simulink model "sschdlexThreePhaseRectifierExample"  (R2023b)
settings: Solver=FixedStepDiscrete  StartTime=0.0  StopTime=0.025  RelTol=1e-6  AbsTol=1e-6
libraries: fl_lib x19, nesl_utility x11
settings Model: DataTypeOverride=Off  Creator=The MathWorks, Inc.  LastModifiedBy=The MathWorks, Inc.
settings SolverCC: AutoScaleAbsTol=off  AlgebraicLoopSolver=TrustRegion
settings DataIOCC: SaveOutput=off  SignalLogging=off  DSMLogging=off  SaveTime=off  ReturnWorkspaceOutputs=off
settings OptimizationCC: BlockReduction=off  ConditionallyExecuteInputs=off  DefaultParameterBehavior=Inlined
settings DebuggingCC: AlgebraicLoopMsg=error  SingleTaskRateTransMsg=error  UnconnectedInputMsg=warning  UnconnectedOutputMsg=warning  UnconnectedLineMsg=warning  PregeneratedLibrarySubsystemCodeDiagnostic=none  ArithmeticOperatorsInVariantConditions=warning
settings HardwareCC: ProdBitPerPointer=32  ProdBitPerSizeT=32  ProdBitPerPtrDiffT=32  ProdLargestAtomicFloat=None  ProdIntDivRoundTo=Undefined  ProdEndianess=Unspecified  ProdWordSize=32  ProdHWDeviceType=ASIC/FPGA->ASIC/FPGA  TargetBitPerPointer=64  TargetBitPerSizeT=64  TargetBitPerPtrDiffT=64  TargetLongLongMode=on  TargetIntDivRoundTo=Zero  TargetEndianess=LittleEndian  TargetWordSize=64  TargetHWDeviceType=Custom Processor->MATLAB Host Computer  ProdEqTarget=off
settings ModelReferenceCC: EnableRefExpFcnMdlSchedulingChecks=on
settings SFSimCC: SimUseLocalCustomCode=off  CustomCodeUndefinedFunction=UseInterfaceOnly
settings RTWCC: RTWUseLocalCustomCode=off
settings CodeAppCC: StateflowObjectComments=on
settings SimscapeCC: SimscapeNormalizeSystem=off  SimscapeNominalValues="[{\"value\":\"10\",\"unit\":\"V\"},{\"value\":\"1\",\"unit\":\"A\"},{\"value\":\"10\",\"unit\":\"N*m\"},{\"value\":\"10\",\"unit\":\"bar\"},{\"value\":\"100\",\"unit\":\"kJ/kg\"},{\"value\":\"1\",\"unit\":\"kW\"},{\"value\":\"300\",\"unit\":\"K\"},{\"value\":\"100\",\"unit\":\"cm^3/s\"},{\"value\":\"1\",\"unit\":\"kN\"},{\"value\":\"1\",\"unit\":\"g/cm^3\"},{\"value\":\"1\",\"unit\":\"l\"},{\"value\":\"1\",\"unit\":\"cm^2\"},{\"value\":\"60\",\"unit\":\"Hz\"}]"  SimscapeLogType=all  SimscapeLogDataHistory=10000

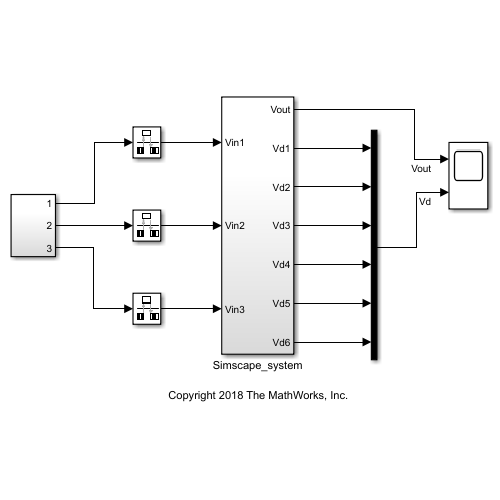
[thumbnail: Simulink's stored preview of the top-level diagram]
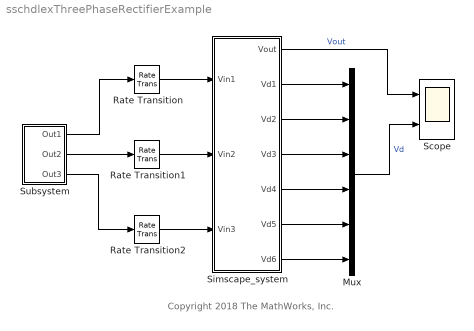
== system sschdlexThreePhaseRectifierExample ==
  note: Copyright 2018 The MathWorks, Inc.
  Mux : Mux  Inputs=6
  Rate Transition : RateTransition
  Rate Transition1 : RateTransition
  Rate Transition2 : RateTransition
  Scope : Scope  NumInputPorts=2
  Simscape_system : Subsystem
  Subsystem : Subsystem
  wires:
  Simscape_system/2(Vd1) -> Mux/1
  Simscape_system/3(Vd2) -> Mux/2
  Simscape_system/4(Vd3) -> Mux/3
  Simscape_system/5(Vd4) -> Mux/4
  Simscape_system/6(Vd5) -> Mux/5
  Simscape_system/7(Vd6) -> Mux/6
  Subsystem/1(Out1) -> Rate Transition/1
  Subsystem/2(Out2) -> Rate Transition1/1
  Subsystem/3(Out3) -> Rate Transition2/1
  Rate Transition/1 -> Simscape_system/1(Vin1)
  Rate Transition1/1 -> Simscape_system/2(Vin2)
  Rate Transition2/1 -> Simscape_system/3(Vin3)
  Simscape_system/1(Vout) -> Scope/1  "Vout"
  Mux/1 -> Scope/2  "Vd"

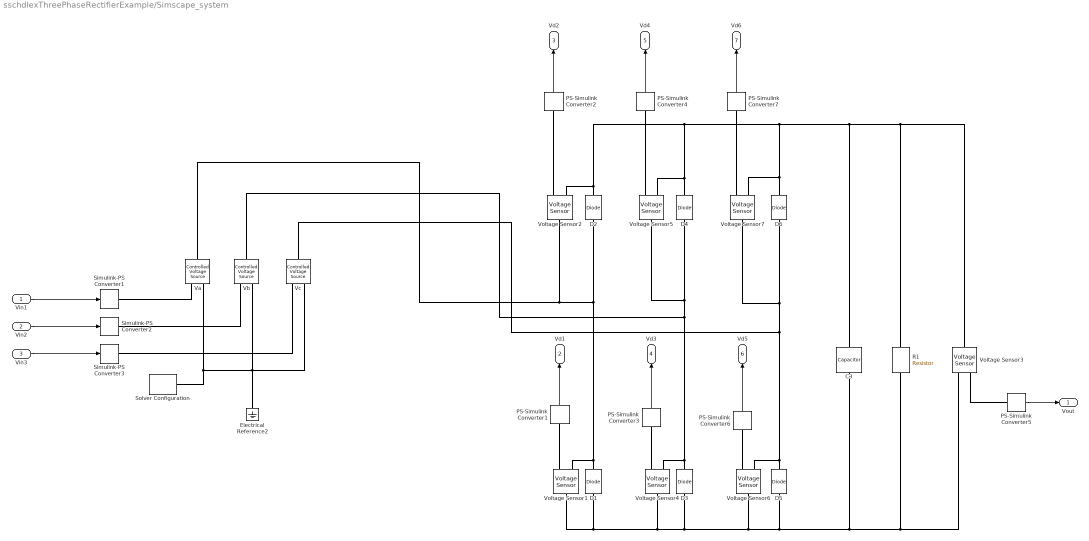
== system sschdlexThreePhaseRectifierExample/Simscape_system ==
  Vin1 : Inport
  Vin2 : Inport  Port=2
  Vin3 : Inport  Port=3
  C3 : fl_lib/Electrical/Electrical Elements/Capacitor  c=10e-3 F  r=1e-6 Ohm  g=0 1/Ohm  i_specify=off  i_priority=None  i=0 A  i_nominal_specify=off  i_nominal_unit=A  i_nominal_value=1  v_specify=off  v_priority=None  v=0 V  v_nominal_specify=off  v_nominal_unit=V  v_nominal_value=1  vc_specify=on  vc_priority=High  vc=150 V  vc_nominal_specify=off  vc_nominal_unit=V  vc_nominal_value=1
  D{1..6} (6 alike) : fl_lib/Electrical/Electrical Elements/Diode  Vf=0.8 V  Ron=0.001 Ohm  Goff=1e-5 1/Ohm  i_specify=off  i_priority=None  i=0 A  i_nominal_specify=off  i_nominal_unit=A  i_nominal_value=1  v_specify=off  v_priority=None  v=0 V  v_nominal_specify=off  v_nominal_unit=V  v_nominal_value=1
  Electrical Reference2 : fl_lib/Electrical/Electrical Elements/Electrical Reference
  PS-Simulink Converter{1..7} (7 alike) : nesl_utility/PS-Simulink Converter  PhysicalDomain=network_engine_domain  SubClassName=ps_output  LeftPortType=input  RightPortType=output  PseudoPeriodic=off  Frequencies=[]  Unit=1  AffineConversion=off
  R1 : fl_lib/Electrical/Electrical Elements/Resistor  R=1 Ohm  i_specify=off  i_priority=None  i=0 A  i_nominal_specify=off  i_nominal_unit=A  i_nominal_value=1  v_specify=off  v_priority=None  v=0 V  v_nominal_specify=off  v_nominal_unit=V  v_nominal_value=1
  Simulink-PS Converter1 : nesl_utility/Simulink-PS Converter  PhysicalDomain=network_engine_domain  SubClassName=ps_input  LeftPortType=input  RightPortType=output  PseudoPeriodic=off  Frequencies=[]  NoiseDistribution=none  NoiseParameters=[]  Unit=1  AffineConversion=off  FilteringAndDerivatives=zero  SimscapeFilterOrder=1  InputFilterTimeConstant=0.001  UdotUserProvided=1
  Simulink-PS Converter2 : nesl_utility/Simulink-PS Converter  PhysicalDomain=network_engine_domain  SubClassName=ps_input  LeftPortType=input  RightPortType=output  PseudoPeriodic=off  Frequencies=[]  NoiseDistribution=none  NoiseParameters=[]  Unit=1  AffineConversion=off  FilteringAndDerivatives=zero  SimscapeFilterOrder=1  InputFilterTimeConstant=0.001  UdotUserProvided=1
  Simulink-PS Converter3 : nesl_utility/Simulink-PS Converter  PhysicalDomain=network_engine_domain  SubClassName=ps_input  LeftPortType=input  RightPortType=output  PseudoPeriodic=off  Frequencies=[]  NoiseDistribution=none  NoiseParameters=[]  Unit=1  AffineConversion=off  FilteringAndDerivatives=zero  SimscapeFilterOrder=1  InputFilterTimeConstant=0.001  UdotUserProvided=1
  Solver Configuration : nesl_utility/Solver Configuration  PhysicalDomain=network_engine_domain  SubClassName=solver  LeftPortType=input  RightPortType=generic  Tones=[]  Harmonics=[]  SimulateNoise=off  Profile=off  UseLocalSampling=off  EnableSwitchedLinearOptims=on  FrequencyDomain=off  UseCCode=off  RelTol=0.001  AbsTol=1e-06  MinStep=1e-09  ToWorkspace=off  RevertToSquareIcSolve=off  NumHomotopyIterations=100  PhasorMode=off  PhasorModeNumHarmonics=1  DoDC=off  ResidualTolerance=1e-09  UseLocalSolver=on  LocalSolverChoice=NE_BACKWARD_EULER_ADVANCER  LocalSolverSampleTime=1e-05  DoFixedCost=off  MaxNonlinIter=3  MaxModeIter=2  LinearAlgebra=Sparse  EquationFormulation=NE_TIME_EF  DelaysMemoryBudget=1024  AutomaticFiltering=on  FilteringTimeConstant=0.001  PartitionStorageMethod=AS_NEEDED  PartitionMemoryBudget=1024
  Va : fl_lib/Electrical/Electrical Sources/Controlled Voltage Source
  Vb : fl_lib/Electrical/Electrical Sources/Controlled Voltage Source
  Vc : fl_lib/Electrical/Electrical Sources/Controlled Voltage Source
  Voltage Sensor{1..7} (7 alike) : fl_lib/Electrical/Electrical Sensors/Voltage Sensor
  Vout : Outport  VectorParamsAs1DForOutWhenUnconnected=off
  Vd1 : Outport  Port=2  VectorParamsAs1DForOutWhenUnconnected=off
  Vd2 : Outport  Port=3  VectorParamsAs1DForOutWhenUnconnected=off
  Vd3 : Outport  Port=4  VectorParamsAs1DForOutWhenUnconnected=off
  Vd4 : Outport  Port=5  VectorParamsAs1DForOutWhenUnconnected=off
  Vd5 : Outport  Port=6  VectorParamsAs1DForOutWhenUnconnected=off
  Vd6 : Outport  Port=7  VectorParamsAs1DForOutWhenUnconnected=off
  wires:
  PS-Simulink Converter5/1 -> Vout/1
  PS-Simulink Converter2/1 -> Vd2/1
  PS-Simulink Converter1/1 -> Vd1/1
  PS-Simulink Converter3/1 -> Vd3/1
  PS-Simulink Converter4/1 -> Vd4/1
  PS-Simulink Converter6/1 -> Vd5/1
  Vin2/1 -> Simulink-PS Converter2/1
  Vin3/1 -> Simulink-PS Converter3/1
  Vin1/1 -> Simulink-PS Converter1/1
  PS-Simulink Converter7/1 -> Vd6/1
  connections:
  PS-Simulink Converter2/LConn1 -- Voltage Sensor2/RConn1
  Vc/LConn1 -- Voltage Sensor7/LConn1 -- D6/LConn1 -- D5/RConn1 -- Voltage Sensor6/RConn2
  Voltage Sensor6/LConn1 -- D1/LConn1 -- Voltage Sensor1/LConn1 -- Voltage Sensor4/LConn1 -- D3/LConn1 -- R1/RConn1 -- Voltage Sensor3/RConn2 -- C3/RConn1 -- D5/LConn1
  D2/LConn1 -- Va/LConn1 -- Voltage Sensor2/LConn1 -- D1/RConn1 -- Voltage Sensor1/RConn2
  C3/LConn1 -- R1/LConn1 -- Voltage Sensor3/LConn1 -- D6/RConn1 -- Voltage Sensor7/RConn2 -- D2/RConn1 -- Voltage Sensor2/RConn2 -- D4/RConn1 -- Voltage Sensor5/RConn2
  PS-Simulink Converter5/LConn1 -- Voltage Sensor3/RConn1
  Va/RConn2 -- Electrical Reference2/LConn1 -- Vb/RConn2 -- Vc/RConn2 -- Solver Configuration/RConn1
  Voltage Sensor5/LConn1 -- D4/LConn1 -- Vb/LConn1 -- D3/RConn1 -- Voltage Sensor4/RConn2
  PS-Simulink Converter1/LConn1 -- Voltage Sensor1/RConn1
  PS-Simulink Converter3/LConn1 -- Voltage Sensor4/RConn1
  PS-Simulink Converter4/LConn1 -- Voltage Sensor5/RConn1
  PS-Simulink Converter6/LConn1 -- Voltage Sensor6/RConn1
  PS-Simulink Converter7/LConn1 -- Voltage Sensor7/RConn1
  Simulink-PS Converter3/RConn1 -- Vc/RConn1
  Simulink-PS Converter2/RConn1 -- Vb/RConn1
  Simulink-PS Converter1/RConn1 -- Va/RConn1

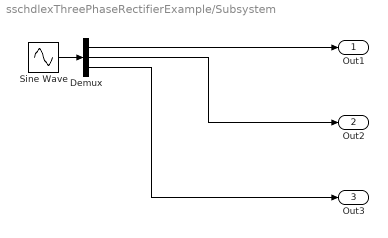
== system sschdlexThreePhaseRectifierExample/Subsystem ==
  Demux : Demux  Outputs=3
  Sine Wave : Sin  Amplitude=100  Frequency=60*2*pi  Phase=[0 -2*pi/3 2*pi/3]  SampleTime=0
  Out1 : Outport  VectorParamsAs1DForOutWhenUnconnected=off
  Out2 : Outport  Port=2  VectorParamsAs1DForOutWhenUnconnected=off
  Out3 : Outport  Port=3  VectorParamsAs1DForOutWhenUnconnected=off
  wires:
  Sine Wave/1 -> Demux/1
  Demux/1 -> Out1/1
  Demux/2 -> Out2/1
  Demux/3 -> Out3/1
